simulink model "GenerateTrajectory"  (R2020b)
settings: Solver=VariableStepAuto  StartTime=0.0  StopTime=10  RelTol=1e-3
settings Model: Creator=이해구  LastModifiedBy=이해구

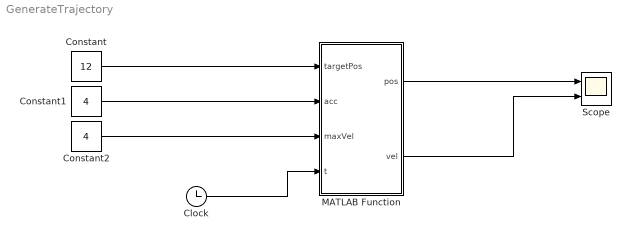
== system GenerateTrajectory ==
  Clock : Clock
  Constant : Constant  Value=12
  Constant1 : Constant  Value=4
  Constant2 : Constant  Value=4
  MATLAB Function : MATLAB Function  TreatAsAtomicUnit=on
  Scope : Scope  NumInputPorts=2
  wires:
  Constant/1 -> MATLAB Function/1(targetPos)
  Constant1/1 -> MATLAB Function/2(acc)
  Constant2/1 -> MATLAB Function/3(maxVel)
  Clock/1 -> MATLAB Function/4(t)
  MATLAB Function/1(pos) -> Scope/1
  MATLAB Function/2(vel) -> Scope/2

== matlab function GenerateTrajectory/MATLAB Function ==
  data: targetPos input; pos output; acc input; maxVel input; vel output; t input
function [pos, vel] = fcn(targetPos, acc, maxVel, t)

ts = 0.004; %4ms
t = 0:ts:5;
posRef = 0;
velRef = 0;

if targetPos > posRef
    velRef = min([(velRef + acc*ts), maxVel, sqrt(2*acc*abs(targetPos-posRef))]);
elseif targetPos < posRef
    velRef = max([(velRef - acc*ts), -maxVel, -sqrt(2*acc*abs(targetPos-posRef))]);            
end
posRef = posRef + velRef*ts;
pos =  posRef;
vel = velRef;
temp
